simulink model "Servo_fn"  (Simulink 7.0)
settings: Solver=ode45  StartTime=0.0  StopTime=10.0  RelTol=1e-3
settings Model: Creator=volgy  LastModifiedBy=Nag

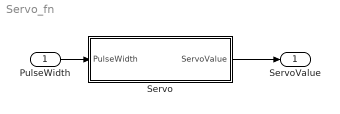
== system Servo_fn ==
  PulseWidth : Inport  OutDataType=sfix(16)  OutScaling=2^0
  Servo : Subsystem
  ServoValue : Outport  OutDataType=sfix(16)  OutScaling=2^0
  wires:
  PulseWidth/1 -> Servo/1(PulseWidth)
  Servo/1(ServoValue) -> ServoValue/1

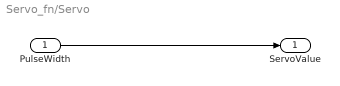
== system Servo_fn/Servo ==
  PulseWidth : Inport  OutDataType=sfix(16)  OutScaling=2^0
  ServoValue : Outport  OutDataType=sfix(16)  OutScaling=2^0
  wires:
  PulseWidth/1 -> ServoValue/1
